simulink model "CartesianImpedanceCtrl"  (R2023b)
settings: Solver=ode45  StartTime=0.0  StopTime=tEnd+5  RelTol=1e-3
undefined symbols (not defined in the file): kinovaGen3, objectPos, q_init, tEnd, Ts, tStart, X, Y, Z
libraries: sm_lib x87, nesl_utility x51, matrix_library x4, robotcorelib x2, robotmaniplib x2, simulink x1
(part 3 of 3)

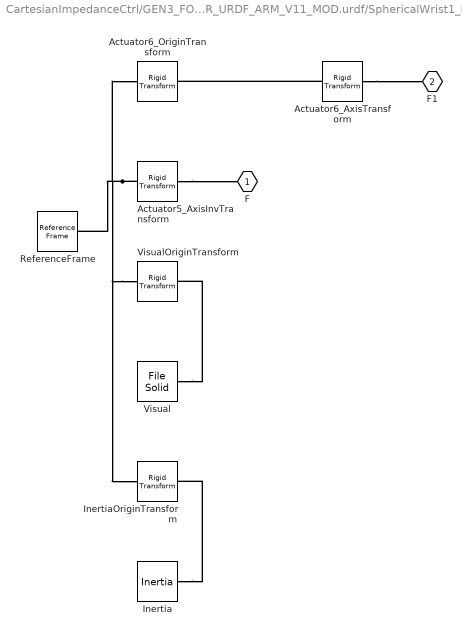
== system CartesianImpedanceCtrl/GEN3_FOR_URDF_ARM_V11_MOD.urdf/SphericalWrist1_Link ==
  Actuator5_AxisInvTransform : sm_lib/Frames and Transforms/Rigid Transform  TranslationMethod=Cartesian  TranslationStandardOffset=0  TranslationStandardOffsetUnits=m  TranslationStandardAxis=+Z  TranslationCartesianOffset=[0, 0, 0]  TranslationCartesianOffsetUnits=m  TranslationROffset=0  TranslationROffsetUnits=m  TranslationZOffset=0  TranslationZOffsetUnits=m  TranslationThetaOffset=0  TranslationThetaOffsetUnits=deg  RotationMethod=ArbitraryAxis  RotationAngleUnits=rad  RotationStandardAxis=+Z  RotationAngle=0  RotationArbitraryAxis=[1, 0, 0]  FollAlignAxisA=+X  BaseAlignAxisA=+Y  FollAlignAxisB=+Y  BaseAlignAxisB=+Z  RotationSequenceAxes=FollowerAxes  RotationSequence=XYX  RotationSequenceAngles=[0 0 0]  RotationSequenceAnglesUnits=deg  RotationMatrix=[1 0 0; 0 1 0; 0 0 1]  Quaternion=[1 0 0 0]
  Actuator6_AxisTransform : sm_lib/Frames and Transforms/Rigid Transform  TranslationMethod=Cartesian  TranslationStandardOffset=0  TranslationStandardOffsetUnits=m  TranslationStandardAxis=+Z  TranslationCartesianOffset=[0, 0, 0]  TranslationCartesianOffsetUnits=m  TranslationROffset=0  TranslationROffsetUnits=m  TranslationZOffset=0  TranslationZOffsetUnits=m  TranslationThetaOffset=0  TranslationThetaOffsetUnits=deg  RotationMethod=ArbitraryAxis  RotationAngleUnits=rad  RotationStandardAxis=+Z  RotationAngle=0  RotationArbitraryAxis=[1, 0, 0]  FollAlignAxisA=+X  BaseAlignAxisA=+Y  FollAlignAxisB=+Y  BaseAlignAxisB=+Z  RotationSequenceAxes=FollowerAxes  RotationSequence=XYX  RotationSequenceAngles=[0 0 0]  RotationSequenceAnglesUnits=deg  RotationMatrix=[1 0 0; 0 1 0; 0 0 1]  Quaternion=[1 0 0 0]
  Actuator6_OriginTransform : sm_lib/Frames and Transforms/Rigid Transform  TranslationMethod=Cartesian  TranslationStandardOffset=0  TranslationStandardOffsetUnits=m  TranslationStandardAxis=+Z  TranslationCartesianOffset=[0, 0.00017505, -0.10593]  TranslationCartesianOffsetUnits=m  TranslationROffset=0  TranslationROffsetUnits=m  TranslationZOffset=0  TranslationZOffsetUnits=m  TranslationThetaOffset=0  TranslationThetaOffsetUnits=deg  RotationMethod=RotationSequence  RotationAngleUnits=deg  RotationStandardAxis=+Z  RotationAngle=0.0  RotationArbitraryAxis=[0 0 1]  FollAlignAxisA=+X  BaseAlignAxisA=+Y  FollAlignAxisB=+Y  BaseAlignAxisB=+Z  RotationSequenceAxes=BaseAxes  RotationSequence=XYZ  RotationSequenceAngles=[1.5708, 3.3255e-17, -8.096199999999999e-15]  RotationSequenceAnglesUnits=rad  RotationMatrix=[1 0 0; 0 1 0; 0 0 1]  Quaternion=[1 0 0 0]
  Inertia : sm_lib/Body Elements/Inertia  InertiaType=Custom  Mass=0.678106  MassUnits=kg  CenterOfMass=[0, 0, 0]  CenterOfMassUnits=m  MomentsOfInertia=[0.001596, 0.001607, 0.000399]  MomentsOfInertiaUnits=kg*m^2  ProductsOfInertia=[0.000256, 0, 0]  ProductsOfInertiaUnits=kg*m^2  GraphicType=None  MarkerShape=Inertia  MarkerSize=20  GraphicVisPropType=SimpleVisualProperties  GraphicDiffuseColor=[0.5 0.5 0.5]  GraphicSpecularColor=[0.5 0.5 0.5 1.0]  GraphicAmbientColor=[0.15 0.15 0.15 1.0]  GraphicEmissiveColor=[0.0 0.0 0.0 1.0]  GraphicShininess=75  GraphicOpacity=1.0
  InertiaOriginTransform : sm_lib/Frames and Transforms/Rigid Transform  TranslationMethod=Cartesian  TranslationStandardOffset=0  TranslationStandardOffsetUnits=m  TranslationStandardAxis=+Z  TranslationCartesianOffset=[1e-06, -0.009431999999999999, -0.063883]  TranslationCartesianOffsetUnits=m  TranslationROffset=0  TranslationROffsetUnits=m  TranslationZOffset=0  TranslationZOffsetUnits=m  TranslationThetaOffset=0  TranslationThetaOffsetUnits=deg  RotationMethod=RotationSequence  RotationAngleUnits=deg  RotationStandardAxis=+Z  RotationAngle=0.0  RotationArbitraryAxis=[0 0 1]  FollAlignAxisA=+X  BaseAlignAxisA=+Y  FollAlignAxisB=+Y  BaseAlignAxisB=+Z  RotationSequenceAxes=BaseAxes  RotationSequence=XYZ  RotationSequenceAngles=[0, 0, 0]  RotationSequenceAnglesUnits=rad  RotationMatrix=[1 0 0; 0 1 0; 0 0 1]  Quaternion=[1 0 0 0]
  ReferenceFrame : sm_lib/Frames and Transforms/Reference Frame
  Visual : sm_lib/Body Elements/File Solid  ExtGeomFileName=GEN3_FOR_URDF_ARM_V11_MOD/meshes/SphericalWrist1_Link.STL  UnitType=Custom  ExtGeomFileUnits=m  StepReaderType=HEX  ExportConvexHullGeometry=off  InertiaType=Custom  Mass=0  MassUnits=kg  CenterOfMass=[0, 0, 0]  CenterOfMassUnits=m  MomentsOfInertia=[0, 0, 0]  MomentsOfInertiaUnits=kg*m^2  ProductsOfInertia=[0, 0, 0]  ProductsOfInertiaUnits=kg*m^2  BasedOnType=DensityFromFile  Density=1000  DensityUnits=kg/m^3  DoExposeReferenceFrame=on  SerializedFrames=<Frames/>  GraphicType=FromGeometry  MarkerShape=Sphere  MarkerSize=10  GraphicVisPropType=SimpleVisualProperties  GraphicDiffuseColor=[0.9569, 0.7529, 0.7529]  GraphicSpecularColor=[0.5 0.5 0.5 1.0]  GraphicAmbientColor=[0.15 0.15 0.15 1.0]  GraphicEmissiveColor=[0.0 0.0 0.0 1.0]  GraphicShininess=75  GraphicOpacity=1
  VisualOriginTransform : sm_lib/Frames and Transforms/Rigid Transform  TranslationMethod=Cartesian  TranslationStandardOffset=0  TranslationStandardOffsetUnits=m  TranslationStandardAxis=+Z  TranslationCartesianOffset=[0, 0, 0]  TranslationCartesianOffsetUnits=m  TranslationROffset=0  TranslationROffsetUnits=m  TranslationZOffset=0  TranslationZOffsetUnits=m  TranslationThetaOffset=0  TranslationThetaOffsetUnits=deg  RotationMethod=RotationSequence  RotationAngleUnits=deg  RotationStandardAxis=+Z  RotationAngle=0.0  RotationArbitraryAxis=[0 0 1]  FollAlignAxisA=+X  BaseAlignAxisA=+Y  FollAlignAxisB=+Y  BaseAlignAxisB=+Z  RotationSequenceAxes=BaseAxes  RotationSequence=XYZ  RotationSequenceAngles=[0, 0, 0]  RotationSequenceAnglesUnits=rad  RotationMatrix=[1 0 0; 0 1 0; 0 0 1]  Quaternion=[1 0 0 0]
  F : PMIOPort  Side=Left
  F1 : PMIOPort  Port=2  Side=Right
  connections:
  Visual/RConn1 -- VisualOriginTransform/RConn1
  VisualOriginTransform/LConn1 -- ReferenceFrame/RConn1 -- InertiaOriginTransform/LConn1 -- Actuator5_AxisInvTransform/LConn1 -- Actuator6_OriginTransform/LConn1
  Inertia/RConn1 -- InertiaOriginTransform/RConn1
  Actuator6_AxisTransform/LConn1 -- Actuator6_OriginTransform/RConn1
  Actuator6_AxisTransform/RConn1 -- F1/RConn1
  Actuator5_AxisInvTransform/RConn1 -- F/RConn1

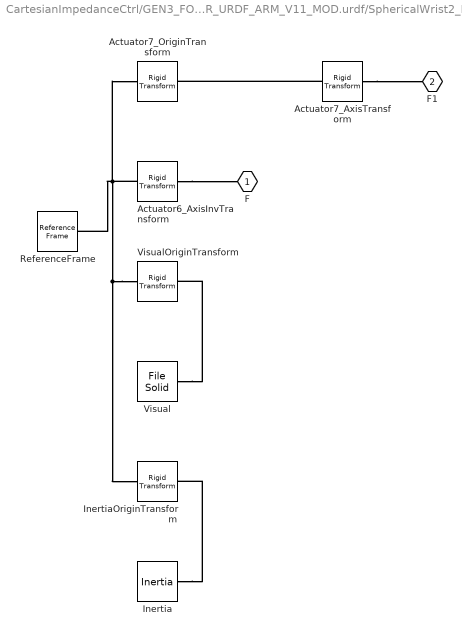
== system CartesianImpedanceCtrl/GEN3_FOR_URDF_ARM_V11_MOD.urdf/SphericalWrist2_Link ==
  Actuator6_AxisInvTransform : sm_lib/Frames and Transforms/Rigid Transform  TranslationMethod=Cartesian  TranslationStandardOffset=0  TranslationStandardOffsetUnits=m  TranslationStandardAxis=+Z  TranslationCartesianOffset=[0, 0, 0]  TranslationCartesianOffsetUnits=m  TranslationROffset=0  TranslationROffsetUnits=m  TranslationZOffset=0  TranslationZOffsetUnits=m  TranslationThetaOffset=0  TranslationThetaOffsetUnits=deg  RotationMethod=ArbitraryAxis  RotationAngleUnits=rad  RotationStandardAxis=+Z  RotationAngle=0  RotationArbitraryAxis=[1, 0, 0]  FollAlignAxisA=+X  BaseAlignAxisA=+Y  FollAlignAxisB=+Y  BaseAlignAxisB=+Z  RotationSequenceAxes=FollowerAxes  RotationSequence=XYX  RotationSequenceAngles=[0 0 0]  RotationSequenceAnglesUnits=deg  RotationMatrix=[1 0 0; 0 1 0; 0 0 1]  Quaternion=[1 0 0 0]
  Actuator7_AxisTransform : sm_lib/Frames and Transforms/Rigid Transform  TranslationMethod=Cartesian  TranslationStandardOffset=0  TranslationStandardOffsetUnits=m  TranslationStandardAxis=+Z  TranslationCartesianOffset=[0, 0, 0]  TranslationCartesianOffsetUnits=m  TranslationROffset=0  TranslationROffsetUnits=m  TranslationZOffset=0  TranslationZOffsetUnits=m  TranslationThetaOffset=0  TranslationThetaOffsetUnits=deg  RotationMethod=ArbitraryAxis  RotationAngleUnits=rad  RotationStandardAxis=+Z  RotationAngle=0  RotationArbitraryAxis=[1, 0, 0]  FollAlignAxisA=+X  BaseAlignAxisA=+Y  FollAlignAxisB=+Y  BaseAlignAxisB=+Z  RotationSequenceAxes=FollowerAxes  RotationSequence=XYX  RotationSequenceAngles=[0 0 0]  RotationSequenceAnglesUnits=deg  RotationMatrix=[1 0 0; 0 1 0; 0 0 1]  Quaternion=[1 0 0 0]
  Actuator7_OriginTransform : sm_lib/Frames and Transforms/Rigid Transform  TranslationMethod=Cartesian  TranslationStandardOffset=0  TranslationStandardOffsetUnits=m  TranslationStandardAxis=+Z  TranslationCartesianOffset=[0, -0.10593, -0.00017505]  TranslationCartesianOffsetUnits=m  TranslationROffset=0  TranslationROffsetUnits=m  TranslationZOffset=0  TranslationZOffsetUnits=m  TranslationThetaOffset=0  TranslationThetaOffsetUnits=deg  RotationMethod=RotationSequence  RotationAngleUnits=deg  RotationStandardAxis=+Z  RotationAngle=0.0  RotationArbitraryAxis=[0 0 1]  FollAlignAxisA=+X  BaseAlignAxisA=+Y  FollAlignAxisB=+Y  BaseAlignAxisB=+Z  RotationSequenceAxes=BaseAxes  RotationSequence=XYZ  RotationSequenceAngles=[-1.5708, -2.3419e-17, 1.52e-17]  RotationSequenceAnglesUnits=rad  RotationMatrix=[1 0 0; 0 1 0; 0 0 1]  Quaternion=[1 0 0 0]
  Inertia : sm_lib/Body Elements/Inertia  InertiaType=Custom  Mass=0.678106  MassUnits=kg  CenterOfMass=[0, 0, 0]  CenterOfMassUnits=m  MomentsOfInertia=[0.001641, 0.00041, 0.001641]  MomentsOfInertiaUnits=kg*m^2  ProductsOfInertia=[-0.000278, 0, 0]  ProductsOfInertiaUnits=kg*m^2  GraphicType=None  MarkerShape=Inertia  MarkerSize=20  GraphicVisPropType=SimpleVisualProperties  GraphicDiffuseColor=[0.5 0.5 0.5]  GraphicSpecularColor=[0.5 0.5 0.5 1.0]  GraphicAmbientColor=[0.15 0.15 0.15 1.0]  GraphicEmissiveColor=[0.0 0.0 0.0 1.0]  GraphicShininess=75  GraphicOpacity=1.0
  InertiaOriginTransform : sm_lib/Frames and Transforms/Rigid Transform  TranslationMethod=Cartesian  TranslationStandardOffset=0  TranslationStandardOffsetUnits=m  TranslationStandardAxis=+Z  TranslationCartesianOffset=[1e-06, -0.045483, -0.009650000000000001]  TranslationCartesianOffsetUnits=m  TranslationROffset=0  TranslationROffsetUnits=m  TranslationZOffset=0  TranslationZOffsetUnits=m  TranslationThetaOffset=0  TranslationThetaOffsetUnits=deg  RotationMethod=RotationSequence  RotationAngleUnits=deg  RotationStandardAxis=+Z  RotationAngle=0.0  RotationArbitraryAxis=[0 0 1]  FollAlignAxisA=+X  BaseAlignAxisA=+Y  FollAlignAxisB=+Y  BaseAlignAxisB=+Z  RotationSequenceAxes=BaseAxes  RotationSequence=XYZ  RotationSequenceAngles=[0, 0, 0]  RotationSequenceAnglesUnits=rad  RotationMatrix=[1 0 0; 0 1 0; 0 0 1]  Quaternion=[1 0 0 0]
  ReferenceFrame : sm_lib/Frames and Transforms/Reference Frame
  Visual : sm_lib/Body Elements/File Solid  ExtGeomFileName=GEN3_FOR_URDF_ARM_V11_MOD/meshes/SphericalWrist2_Link.STL  UnitType=Custom  ExtGeomFileUnits=m  StepReaderType=HEX  ExportConvexHullGeometry=off  InertiaType=Custom  Mass=0  MassUnits=kg  CenterOfMass=[0, 0, 0]  CenterOfMassUnits=m  MomentsOfInertia=[0, 0, 0]  MomentsOfInertiaUnits=kg*m^2  ProductsOfInertia=[0, 0, 0]  ProductsOfInertiaUnits=kg*m^2  BasedOnType=DensityFromFile  Density=1000  DensityUnits=kg/m^3  DoExposeReferenceFrame=on  SerializedFrames=<Frames/>  GraphicType=FromGeometry  MarkerShape=Sphere  MarkerSize=10  GraphicVisPropType=SimpleVisualProperties  GraphicDiffuseColor=[0.9216, 0.949, 0.7647]  GraphicSpecularColor=[0.5 0.5 0.5 1.0]  GraphicAmbientColor=[0.15 0.15 0.15 1.0]  GraphicEmissiveColor=[0.0 0.0 0.0 1.0]  GraphicShininess=75  GraphicOpacity=1
  VisualOriginTransform : sm_lib/Frames and Transforms/Rigid Transform  TranslationMethod=Cartesian  TranslationStandardOffset=0  TranslationStandardOffsetUnits=m  TranslationStandardAxis=+Z  TranslationCartesianOffset=[0, 0, 0]  TranslationCartesianOffsetUnits=m  TranslationROffset=0  TranslationROffsetUnits=m  TranslationZOffset=0  TranslationZOffsetUnits=m  TranslationThetaOffset=0  TranslationThetaOffsetUnits=deg  RotationMethod=RotationSequence  RotationAngleUnits=deg  RotationStandardAxis=+Z  RotationAngle=0.0  RotationArbitraryAxis=[0 0 1]  FollAlignAxisA=+X  BaseAlignAxisA=+Y  FollAlignAxisB=+Y  BaseAlignAxisB=+Z  RotationSequenceAxes=BaseAxes  RotationSequence=XYZ  RotationSequenceAngles=[0, 0, 0]  RotationSequenceAnglesUnits=rad  RotationMatrix=[1 0 0; 0 1 0; 0 0 1]  Quaternion=[1 0 0 0]
  F : PMIOPort  Side=Left
  F1 : PMIOPort  Port=2  Side=Right
  connections:
  Visual/RConn1 -- VisualOriginTransform/RConn1
  VisualOriginTransform/LConn1 -- Actuator6_AxisInvTransform/LConn1 -- ReferenceFrame/RConn1 -- Actuator7_OriginTransform/LConn1 -- InertiaOriginTransform/LConn1
  Inertia/RConn1 -- InertiaOriginTransform/RConn1
  Actuator7_AxisTransform/LConn1 -- Actuator7_OriginTransform/RConn1
  Actuator7_AxisTransform/RConn1 -- F1/RConn1
  Actuator6_AxisInvTransform/RConn1 -- F/RConn1

== system CartesianImpedanceCtrl/GEN3_FOR_URDF_ARM_V11_MOD.urdf/Subsystem ==
  MATLAB Function1 : MATLAB Function  TreatAsAtomicUnit=on
  PS-Simulink Converter{3..6} (4 alike) : nesl_utility/PS-Simulink Converter  PhysicalDomain=network_engine_domain  SubClassName=ps_output  LeftPortType=input  RightPortType=output  PseudoPeriodic=off  Frequencies=[]  VectorFormat=1-D array  Unit=inherit  AffineConversion=off
  Transform Sensor1 : sm_lib/Frames and Transforms/Transform Sensor  MeasurementFrame=World  RotationSequence=XYX  SenseAngle=off  SenseAxis=off  SenseQ=off  SenseR=on  SenseRotationSequence=off  SenseOmegaX=off  SenseOmegaY=off  SenseOmegaZ=off  SenseOmega=off  SenseQDot=off  SenseRDot=off  SenseRotationSequenceDot=off  SenseAlphaX=off  SenseAlphaY=off  SenseAlphaZ=off  SenseAlpha=off  SenseQDDot=off  SenseRDDot=off  SenseX=on  SenseY=on  SenseZ=on  SenseXYZ=off  SenseRad=off  SenseAzim=off  SenseDist=off  SenseInc=off  SenseXDot=off  SenseYDot=off  SenseZDot=off  SenseXYZDot=off  SenseRadDot=off  SenseAzimDot=off  SenseDistDot=off  SenseIncDot=off  SenseXDDot=off  SenseYDDot=off  SenseZDDot=off  SenseXYZDDot=off  SenseRadDDot=off  SenseAzimDDot=off  SenseDistDDot=off  SenseIncDDot=off
  Conn1 : PMIOPort  Side=Left
  Obstacle1 : PMIOPort  Port=2  Side=Right
  Contact Points Transform : Outport
  wires:
  PS-Simulink Converter5/1 -> MATLAB Function1/3(y)
  PS-Simulink Converter3/1 -> MATLAB Function1/1(R)
  PS-Simulink Converter6/1 -> MATLAB Function1/4(z)
  PS-Simulink Converter4/1 -> MATLAB Function1/2(x)
  MATLAB Function1/1(T) -> Contact Points Transform/1
  connections:
  Transform Sensor1/RConn3 -- PS-Simulink Converter4/LConn1
  Transform Sensor1/RConn2 -- PS-Simulink Converter3/LConn1
  Transform Sensor1/RConn4 -- PS-Simulink Converter5/LConn1
  Transform Sensor1/RConn5 -- PS-Simulink Converter6/LConn1
  Transform Sensor1/LConn1 -- Conn1/RConn1
  Transform Sensor1/RConn1 -- Obstacle1/RConn1

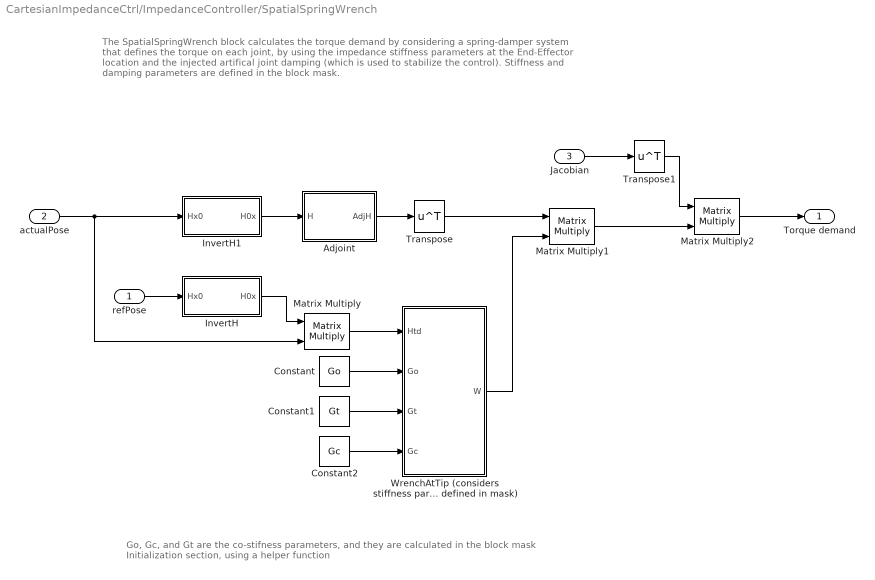
== system CartesianImpedanceCtrl/ImpedanceController/SpatialSpringWrench ==
  note: The SpatialSpringWrench block calculates the torque demand by considering a spring-damper system that defines the torque on each joint, by using the impedance stiffness parameters at the End-Effector location and the injected artifical joint damping (which is used to stabilize the control). Stiffness and damping parameters are defined in the block mask.
  note: Go, Gc, and Gt are the co-stifness parameters, and they are calculated in the block mask Initialization section, using a helper function
  refPose : Inport
  actualPose : Inport  Port=2
  Jacobian : Inport  Port=3
  Adjoint : MATLAB Function  TreatAsAtomicUnit=on
  Constant : Constant  Value=Go
  Constant1 : Constant  Value=Gt
  Constant2 : Constant  Value=Gc
  InvertH : Subsystem
  InvertH1 : Subsystem
  Matrix Multiply : Product  Multiplication=Matrix(*)
  Matrix Multiply1 : Product  Multiplication=Matrix(*)
  Matrix Multiply2 : Product  Multiplication=Matrix(*)
  Transpose : Math  Operator=transpose
  Transpose1 : Math  Operator=transpose
  WrenchAtTip (considers stiffness parameters defined in mask) : MATLAB Function  TreatAsAtomicUnit=on
  Torque demand : Outport
  wires:
  Constant2/1 -> WrenchAtTip (considers stiffness parameters defined in mask)/4(Gc)
  Constant1/1 -> WrenchAtTip (considers stiffness parameters defined in mask)/3(Gt)
  Constant/1 -> WrenchAtTip (considers stiffness parameters defined in mask)/2(Go)
  Matrix Multiply2/1 -> Torque demand/1
  Transpose1/1 -> Matrix Multiply2/1
  Jacobian/1 -> Transpose1/1
  Matrix Multiply1/1 -> Matrix Multiply2/2
  WrenchAtTip (considers stiffness parameters defined in mask)/1(W) -> Matrix Multiply1/2
  Transpose/1 -> Matrix Multiply1/1
  InvertH1/1(H0x) -> Adjoint/1(H)
  Matrix Multiply/1 -> WrenchAtTip (considers stiffness parameters defined in mask)/1(Htd)
  refPose/1 -> InvertH/1(Hx0)
  InvertH/1(H0x) -> Matrix Multiply/1
  actualPose/1 -> Matrix Multiply/2, InvertH1/1(Hx0)
  Adjoint/1(AdjH) -> Transpose/1

== system CartesianImpedanceCtrl/ImpedanceController/Unwrap Position-Velocity (PV) to Joint q-dq ==
  PV : Inport
  Bus Selector : BusSelector  OutputSignals=J1.q,J2.q,J3.q,J4.q,J5.q,J6.q,J7.q
  Bus Selector1 : BusSelector  OutputSignals=J1.w,J2.w,J3.w,J4.w,J5.w,J6.w,J7.w
  Mux : Mux  Inputs=7
  Mux1 : Mux  Inputs=7
  q : Outport
  dq : Outport  Port=2
  wires:
  Mux1/1 -> dq/1
  Bus Selector1/4 -> Mux1/4  "<w>"
  Bus Selector1/7 -> Mux1/7  "<w>"
  Bus Selector/3 -> Mux/3  "<q>"
  Bus Selector/6 -> Mux/6  "<q>"
  Bus Selector/7 -> Mux/7  "<q>"
  Bus Selector1/2 -> Mux1/2  "<w>"
  Bus Selector/2 -> Mux/2  "<q>"
  Bus Selector1/5 -> Mux1/5  "<w>"
  Bus Selector/5 -> Mux/5  "<q>"
  Bus Selector1/6 -> Mux1/6  "<w>"
  Bus Selector/1 -> Mux/1  "<q>"
  Bus Selector1/1 -> Mux1/1  "<w>"
  Mux/1 -> q/1
  PV/1 -> Bus Selector1/1, Bus Selector/1
  Bus Selector1/3 -> Mux1/3  "<w>"
  Bus Selector/4 -> Mux/4  "<q>"

== system CartesianImpedanceCtrl/Obstacle/Wall Object ==
  Inertia : sm_lib/Body Elements/Brick Solid  GraphicAmbientColor=[0.15 0.15 0.15 1.0]  BasedOnType=Density  BrickDimensions=[0.1 1 1]  BrickDimensionsUnits=m  CenterOfMass=[0, 0, 0]  CenterOfMassUnits=m  GraphicDiffuseColor=[0.6 0.8 1.0]  Density=1000  DensityUnits=kg/m^3  DoExposeReferenceFrame=on  GraphicEmissiveColor=[0.0 0.0 0.0 1.0]  ExportEntireGeometry=on  SerializedFrames=<Frames/>  MarkerShape=Sphere  MarkerSize=10  GraphicType=FromGeometry  InertiaType=Custom  Mass=1e8  MassUnits=kg  MomentsOfInertia=[1e-08, 1e-08, 1e-08]  MomentsOfInertiaUnits=kg*m^2  GraphicOpacity=0.5  ProductsOfInertia=[1e-08, 1e-08, 1e-08]  ProductsOfInertiaUnits=kg*m^2  GraphicShininess=75  GraphicSpecularColor=[0.5 0.5 0.5 1.0]  GraphicVisPropType=SimpleVisualProperties
  InertiaOriginTransform : sm_lib/Frames and Transforms/Rigid Transform  TranslationMethod=Cartesian  TranslationStandardOffset=0  TranslationStandardOffsetUnits=m  TranslationStandardAxis=+Z  TranslationCartesianOffset=[1e-08, 1e-08, 0.5]  TranslationCartesianOffsetUnits=m  TranslationROffset=0  TranslationROffsetUnits=m  TranslationZOffset=0  TranslationZOffsetUnits=m  TranslationThetaOffset=0  TranslationThetaOffsetUnits=deg  RotationMethod=RotationSequence  RotationAngleUnits=deg  RotationStandardAxis=+Z  RotationAngle=0.0  RotationArbitraryAxis=[0 0 1]  FollAlignAxisA=+X  BaseAlignAxisA=+Y  FollAlignAxisB=+Y  BaseAlignAxisB=+Z  RotationSequenceAxes=BaseAxes  RotationSequence=XYZ  RotationSequenceAngles=[0, 0, 0]  RotationSequenceAnglesUnits=rad  RotationMatrix=[1 0 0; 0 1 0; 0 0 1]  Quaternion=[1 0 0 0]
  ReferenceFrame : sm_lib/Frames and Transforms/Reference Frame
  F : PMIOPort  Side=Left
  Obstacle Geometry : PMIOPort  Port=2  Side=Right
  connections:
  Obstacle Geometry/RConn1 -- Inertia/LConn1
  F/RConn1 -- InertiaOriginTransform/LConn1 -- ReferenceFrame/RConn1
  Inertia/RConn1 -- InertiaOriginTransform/RConn1

== system CartesianImpedanceCtrl/ImpedanceController/SpatialSpringWrench/InvertH ==
  Hx0 : Inport
  Constant : Constant  Value=[0 0 0 1]  VectorParams1D=off
  Gain : Gain  Gain=-1
  Matrix Concatenate : Concatenate  Mode=Multidimensional array  ConcatenateDimension=2
  Matrix Concatenate1 : Concatenate  Mode=Multidimensional array
  Matrix Multiply : Product  Multiplication=Matrix(*)
  Submatrix : matrix_library/Submatrix  RowSpan=Range of rows  RowStartMode=First  RowStartIndex=1  RowEndMode=Index  RowEndIndex=3  ColSpan=Range of columns  ColStartMode=First  ColStartIndex=1  ColEndMode=Index  ColEndIndex=3
  Submatrix1 : matrix_library/Submatrix  RowSpan=Range of rows  RowStartMode=First  RowStartIndex=1  RowEndMode=Index  RowEndIndex=3  ColSpan=One column  ColStartMode=Last  ColStartIndex=1  ColEndMode=Index  ColEndIndex=3
  Transpose : Math  Operator=transpose
  H0x : Outport
  wires:
  Matrix Concatenate1/1 -> H0x/1
  Matrix Concatenate/1 -> Matrix Concatenate1/1
  Submatrix1/1 -> Matrix Multiply/2
  Matrix Multiply/1 -> Matrix Concatenate/2
  Gain/1 -> Matrix Multiply/1
  Submatrix/1 -> Transpose/1
  Constant/1 -> Matrix Concatenate1/2
  Hx0/1 -> Submatrix/1, Submatrix1/1
  Transpose/1 -> Gain/1, Matrix Concatenate/1

== system CartesianImpedanceCtrl/ImpedanceController/SpatialSpringWrench/InvertH1 ==
  Hx0 : Inport
  Constant : Constant  Value=[0 0 0 1]  VectorParams1D=off
  Gain : Gain  Gain=-1
  Matrix Concatenate : Concatenate  Mode=Multidimensional array  ConcatenateDimension=2
  Matrix Concatenate1 : Concatenate  Mode=Multidimensional array
  Matrix Multiply : Product  Multiplication=Matrix(*)
  Submatrix : matrix_library/Submatrix  RowSpan=Range of rows  RowStartMode=First  RowStartIndex=1  RowEndMode=Index  RowEndIndex=3  ColSpan=Range of columns  ColStartMode=First  ColStartIndex=1  ColEndMode=Index  ColEndIndex=3
  Submatrix1 : matrix_library/Submatrix  RowSpan=Range of rows  RowStartMode=First  RowStartIndex=1  RowEndMode=Index  RowEndIndex=3  ColSpan=One column  ColStartMode=Last  ColStartIndex=1  ColEndMode=Index  ColEndIndex=3
  Transpose : Math  Operator=transpose
  H0x : Outport
  wires:
  Transpose/1 -> Matrix Concatenate/1, Gain/1
  Hx0/1 -> Submatrix1/1, Submatrix/1
  Constant/1 -> Matrix Concatenate1/2
  Submatrix/1 -> Transpose/1
  Gain/1 -> Matrix Multiply/1
  Matrix Multiply/1 -> Matrix Concatenate/2
  Submatrix1/1 -> Matrix Multiply/2
  Matrix Concatenate/1 -> Matrix Concatenate1/1
  Matrix Concatenate1/1 -> H0x/1

== matlab function CartesianImpedanceCtrl/GEN3_FOR_URDF_ARM_V11_MOD.urdf/Subsystem/MATLAB Function1 ==
  data: R input; T output; x input; y input; z input
function T = createHomTransMat(R,x,y,z)

T = eye(4);
T(1:3,1:3) = R;
T(1:3,4) = [x y z]';

== matlab function CartesianImpedanceCtrl/GEN3_FOR_URDF_ARM_V11_MOD.urdf/MATLAB Function ==
  data: vx input; dirVel output; vy input; vz input
function dirVel = findVelDirection(vx,vy,vz)

if norm([vx,vy,vz]) <= eps
    dirVel = [0 0 0];
else
    dirVel = [vx vy vz]/norm([vx,vy,vz]);
end
end

== matlab function CartesianImpedanceCtrl/ImpedanceController/SpatialSpringWrench/Adjoint ==
  data: H input; AdjH output
function AdjH = fcn(H)
%#codegen
R = H(1:3,1:3);
P = H(1:3,4);
AdjH = [     R       zeros(3);
         Tilde(P)*R     R      ];

== matlab function CartesianImpedanceCtrl/ImpedanceController/SpatialSpringWrench/WrenchAtTip (considers stiffness parameters defined in mask) ==
  data: Htd input; W output; Go input; Gt input; Gc input
function W = fcn(Htd, Go, Gt, Gc)
% Calculates End-Effector wrench
%#codegen

% Rotation
Rtd = Htd(1:3,1:3);
% Position
Ptd = Htd(1:3,4);
%Calculate the moment 
Mt = -2*SkSym(Go*Rtd) - SkSym(Gt*Rtd'*Tilde(Ptd)*Tilde(Ptd)*Rtd) - 2*SkSym(Gc*Tilde(Ptd)*Rtd);
M = UnTilde(Mt);
%Calculate the force
Ft = -Rtd'*SkSym(Gt*Tilde(Ptd))*Rtd - SkSym(Gt*Rtd'*Tilde(Ptd)*Rtd) - 2*SkSym(Gc*Rtd);
F = UnTilde(Ft);
% wrench
W = [M;F];

== matlab function CartesianImpedanceCtrl/GEN3_FOR_URDF_ARM_V11_MOD.urdf/MATLAB Function1 ==
  data: fn input; wrenchContact output; ft input; velDir input; T input
function wrenchContact = estimateEEWrench(fn,ft,velDir,T)
%#codegen

%%% Ff = Adj_Taf'*Fa
wrenchContact = calcAdjMatrix(T(1:3,1:3),T(1:3,4))'*[0 0 0 -fn ft*-velDir(2) ft*-velDir(3)]'; 

end

function adjMat = calcAdjMatrix(R,p)
%#codegen
    adjMat = [R zeros(3); calcSkewSymMatrix(p)*R R];
end

function skewSymMat = calcSkewSymMatrix(v)
%#codegen
    x = v(1); y = v(2); z = v(3);
    skewSymMat = [0 -z y ; z 0 -x;-y x 0];
end
